simulink model "Inverse_Kinetic"  (R2020a)
settings: Solver=VariableStepAuto  StartTime=0.0  StopTime=10000  RelTol=1e-3
libraries: simulink x5, roblocks x2
settings Model: EnablePacing=on  Creator=hemingshan  LastModifiedBy=hemingshan

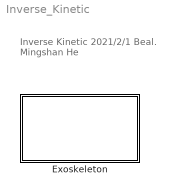
== system Inverse_Kinetic ==
  note: Inverse Kinetic
      | 2021/2/1
      | Beal. Mingshan He
  Exoskeleton : Subsystem
      mask Display: disp('Inverse Kinetic');

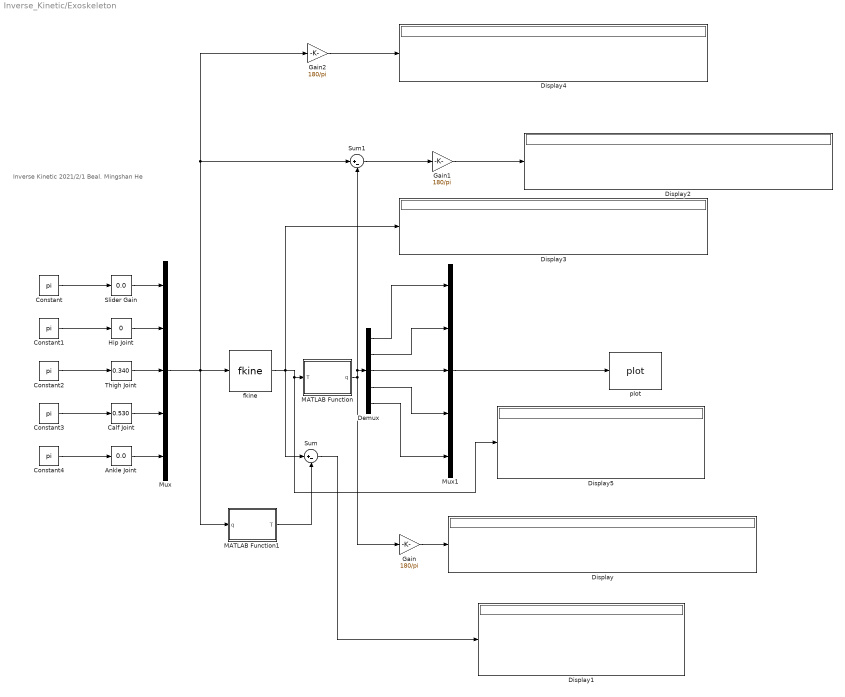
== system Inverse_Kinetic/Exoskeleton ==
  note: Inverse Kinetic
      | 2021/2/1
      | Beal. Mingshan He
  Ankle Joint : simulink/Math Operations/Slider Gain  gain=0.0  low=0  high=0.5
  Calf Joint : simulink/Math Operations/Slider Gain  gain=0.530  low=0  high=1
  Constant{,1..4} (5 alike) : Constant  Value=pi
  Demux : Demux  Outputs=5
  Display{,1..5} (6 alike) : Display
  Gain : Gain  Gain=180/pi
  Gain1 : Gain  Gain=180/pi
  Gain2 : Gain  Gain=180/pi
  Hip Joint : simulink/Math Operations/Slider Gain  gain=0  low=0  high=2
  MATLAB Function : MATLAB Function  TreatAsAtomicUnit=on
  MATLAB Function1 : MATLAB Function  TreatAsAtomicUnit=on
  Mux : Mux  Inputs=5
  Mux1 : Mux  Inputs=5
  Slider Gain : simulink/Math Operations/Slider Gain  gain=0.0  low=0  high=2
  Sum : Sum  Inputs=|+-
  Sum1 : Sum  Inputs=|+-
  Thigh Joint : simulink/Math Operations/Slider Gain  gain=0.340  low=0  high=1
  fkine : roblocks/Arm/fkine  robot=robot
  plot : roblocks/Arm/plot  robot=robot  fps=5  holdplot=on
  wires:
  Gain/1 -> Display/1
  Constant3/1 -> Calf Joint/1
  Mux1/1 -> plot/1
  Demux/3 -> Mux1/3
  MATLAB Function/1(q) -> Sum1/2, Demux/1, Gain/1
  Sum/1 -> Display1/1
  Gain1/1 -> Display2/1
  fkine/1 -> Display3/1, Display5/1, MATLAB Function/1(T), Sum/1
  Demux/2 -> Mux1/2
  Demux/5 -> Mux1/5
  Gain2/1 -> Display4/1
  Sum1/1 -> Gain1/1
  Constant4/1 -> Ankle Joint/1
  Demux/1 -> Mux1/1
  Ankle Joint/1 -> Mux/5
  Hip Joint/1 -> Mux/2
  Mux/1 -> Gain2/1, Sum1/1, fkine/1, MATLAB Function1/1(q)
  Constant2/1 -> Thigh Joint/1
  Demux/4 -> Mux1/4
  Slider Gain/1 -> Mux/1
  Thigh Joint/1 -> Mux/3
  MATLAB Function1/1(T) -> Sum/2
  Calf Joint/1 -> Mux/4
  Constant/1 -> Slider Gain/1
  Constant1/1 -> Hip Joint/1

== matlab function Inverse_Kinetic/Exoskeleton/MATLAB Function ==
  data: T input; q output
function q= fcn(T)
%theta-offset
% offset1 = 0;
% offset2 = pi/2-atan(0.23966/0.28189);
% offset3 = pi/2-atan(0.23966/0.28189)+atan(0.15989/0.31135);
% offset4 = -atan(0.15989/0.31135);
%%DH
d1 = -0.097;
a3 = -sqrt(0.23966^2+0.28189^2);
a4 = -sqrt(-0.15989^2+0.31135^2);
%%theta1
  theta1 = atan2(T(1,3),-T(2,3));
%%theta3
  equ1 = T(1,4)^2 + T(2,4)^2;
  equ2 = (T(3,4)-d1)^2;
  equ3 = equ1 + equ2;
  c3   = (equ3 - a3^2 - a4^2)/(2*a3*a4);
%   s3   = sqrt(1-c3^2);
  if 1-c3^2 < 1e-20
      s3 = 0;
  else
      s3   = sqrt(1-c3^2);
  end
  theta3 = atan2(s3,c3);
  
%%theta2
  
  x = (T(1,4)^2+T(2,4)^2)^0.5;
  y = T(3,4)-d1;
  if T(1,4) < 0
      x = -x;
  end
  k1 = (a4*cos(theta3)+a3);
  k2 = -sin(theta3)*a4;
  theta2 = atan2(y,x)+ atan2(k2,k1);
%   atan = atan2(k2,k1)
%   theta2 = -theta2;
  
%%theta4
  phi = atan2(T(3,1),T(3,2));
  theta4 = phi - theta2 - theta3;
  q = [0,theta1,theta2,theta3,theta4];

== matlab function Inverse_Kinetic/Exoskeleton/MATLAB Function1 ==
  data: q input; T output
function T = fcn(q)
theta1 = q(2);
theta2 = q(3);
theta3 = q(4);
theta4 = q(5);
d1 = -0.097;
a3 = -sqrt(0.23966^2+0.28189^2);
a4 = -sqrt(-0.15989^2+0.31135^2);
Tbase = [1 0 0 0;
         0 1 0 0;
         0 0 1 d1;
         0 0 0 1];
    
T1=[1 0 0 0;
    0 1 0 0;
    0 0 1 0;
    0 0 0 1];

T2=[cos(theta1) -sin(theta1) 0 0;
    sin(theta1)  cos(theta1)  0 0;
    0   0   1 0;
    0   0   0 1];
T3=[cos(theta2) -sin(theta2) 0 0;
    0   0  -1 0;
    sin(theta2)  cos(theta2)  0 0;
    0   0   0 1];
T4=[cos(theta3) -sin(theta3) 0 a3;
    sin(theta3) cos(theta3)  0 0;
    0  0   1 0;
    0  0   0 1];
Ttool = [cos(theta4) -sin(theta4) 0 a4;
         sin(theta4)  cos(theta4) 0 0;
         0    0 1 0;
         0    0 0 1];

T = Tbase*T1*T2*T3*T4*Ttool
